simulink model "Ericc_veleves"  (R2015b)
settings: Solver=ode45  StartTime=0.0  StopTime=1  MaxStep=0.01  RelTol=1e-3
values from neighbouring files (symbols this model uses):
  Cfsec = 1    [para.m]
  DAC = 1    [para.m]
  Kd = 0    [para.m]
  Ki = 0    [para.m]
  Kp = 1000    [para.m]
undefined symbols (not defined in the file or in its folder): Cfesc
settings Model: Creator=antomart  LastModifiedBy=David
settings DataIOCC: LimitDataPoints=off  SaveFormat=StructureWithTime
settings HardwareCC: ProdWordSize=32  ProdHWDeviceType=Specified
settings ModelReferenceCC: PropagateSignalLabelsOutOfModel=on
settings GRTTargetCC: GeneratePreprocessorConditionals=Disable all

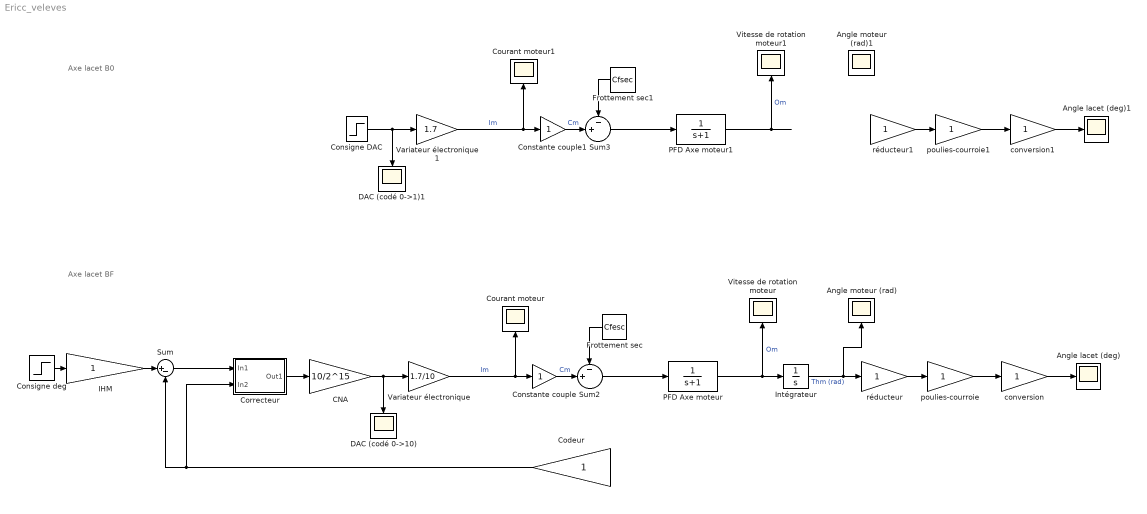
== system Ericc_veleves ==
  note: Axe lacet BF
  note: Axe lacet B0
  Angle moteur (rad) : Scope
  Angle moteur (rad)1 : Scope
  Angle lacet (deg) : Scope
  Angle lacet (deg)1 : Scope
  CNA : Gain  Gain=10/2^15
  Codeur : Gain
  Consigne DAC : Step  Time=0  After=DAC  SampleTime=0
  Consigne deg : Step  Time=0  After=30  SampleTime=0
  Constante couple : Gain
  Constante couple1 : Gain
  Correcteur : Subsystem
  Courant moteur : Scope
  Courant moteur1 : Scope
  DAC (codé 0->1)1 : Scope
  DAC (codé 0->10) : Scope
  Frottement sec : Constant  Value=Cfesc
  Frottement sec1 : Constant  Value=Cfsec
  IHM : Gain
  Intégrateur : Integrator
  PFD Axe moteur : TransferFcn  Denominator=[1 1]
  PFD Axe moteur1 : TransferFcn  Denominator=[1 1]
  Sum : Sum  Inputs=|+-
  Sum2 : Sum  Inputs=-+|
  Sum3 : Sum  Inputs=-+|
  Variateur électronique : Gain  Gain=1.7/10
  Variateur électronique1 : Gain  Gain=1.7
  Vitesse de rotation moteur : Scope
  Vitesse de rotation moteur1 : Scope
  conversion : Gain
  conversion1 : Gain
  poulies-courroie : Gain
  poulies-courroie1 : Gain
  réducteur : Gain
  réducteur1 : Gain
  wires:
  PFD Axe moteur/1 -> Intégrateur/1, Vitesse de rotation moteur/1  "Om"
  Intégrateur/1 -> réducteur/1, Angle moteur (rad)/1  "Thm (rad)"
  réducteur/1 -> poulies-courroie/1
  Sum/1 -> Correcteur/1(In1)
  Correcteur/1(Out1) -> CNA/1
  Consigne deg/1 -> IHM/1
  Codeur/1 -> Correcteur/2(In2), Sum/2
  IHM/1 -> Sum/1
  conversion/1 -> Angle lacet (deg)/1
  Sum2/1 -> PFD Axe moteur/1
  Frottement sec/1 -> Sum2/1
  Constante couple/1 -> Sum2/2  "Cm"
  CNA/1 -> Variateur électronique/1, DAC (codé 0->10)/1
  poulies-courroie/1 -> conversion/1
  Variateur électronique/1 -> Constante couple/1, Courant moteur/1  "Im"
  PFD Axe moteur1/1 -> Vitesse de rotation moteur1/1  "Om"
  ? -> réducteur1/1, Angle moteur (rad)1/1  "Thm (rad)"
  réducteur1/1 -> poulies-courroie1/1
  conversion1/1 -> Angle lacet (deg)1/1
  Sum3/1 -> PFD Axe moteur1/1
  Frottement sec1/1 -> Sum3/1
  Constante couple1/1 -> Sum3/2  "Cm"
  Consigne DAC/1 -> Variateur électronique1/1, DAC (codé 0->1)1/1
  poulies-courroie1/1 -> conversion1/1
  Variateur électronique1/1 -> Constante couple1/1, Courant moteur1/1  "Im"

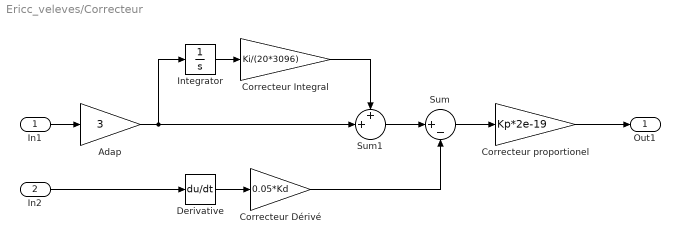
== system Ericc_veleves/Correcteur ==
  In1 : Inport
  In2 : Inport  Port=2
  Adap : Gain  Gain=3
  Correcteur Dérivé : Gain  Gain=0.05*Kd
  Correcteur Integral : Gain  Gain=Ki/(20*3096)
  Correcteur proportionel : Gain  Gain=Kp*2e-19
  Derivative : Derivative
  Integrator : Integrator
  Sum : Sum  Inputs=|+-
  Sum1 : Sum  Inputs=++|
  Out1 : Outport
  wires:
  In1/1 -> Adap/1
  Integrator/1 -> Correcteur Integral/1
  Derivative/1 -> Correcteur Dérivé/1
  Correcteur Dérivé/1 -> Sum/2
  Sum/1 -> Correcteur proportionel/1
  Adap/1 -> Sum1/2, Integrator/1
  Correcteur proportionel/1 -> Out1/1
  In2/1 -> Derivative/1
  Sum1/1 -> Sum/1
  Correcteur Integral/1 -> Sum1/1
